simulink model "pmsm_2dof_control"  (R2018b)
settings: Solver=VariableStepAuto  StartTime=0.0  StopTime=20  RelTol=1e-3
model workspace (MATLAB code in the model file):
  | np=4; % pole pairs
  | phiv=0.1167; % rotor flux, wb
  | Kt=3/2*np*phiv;
  | f=7.43e-5; %Nm/(rad/s), friction
  | J=1.74e-4; %kgm*m, inertia
  | L=0.004; %H, inductance
  | Ld=L;
  | Lq=L;
  | Rs=1.74; %Ohm, armature resistance
  | Kp=50; % Prop gain in inner PI
  | Ki=2500; % I gain in inner PI
  | Ti = Kp/Ki;
  | h = 1e-2; % Sampling period
  | wN = pi/h; % Nyquist freq
  | wBf = 0.7*wN; % Cutoff freq for AA filter
  | w0f = wBf/2.11; % AA filter param
libraries: simulink x1
settings Model: Creator=kjartan  LastModifiedBy=kjartan

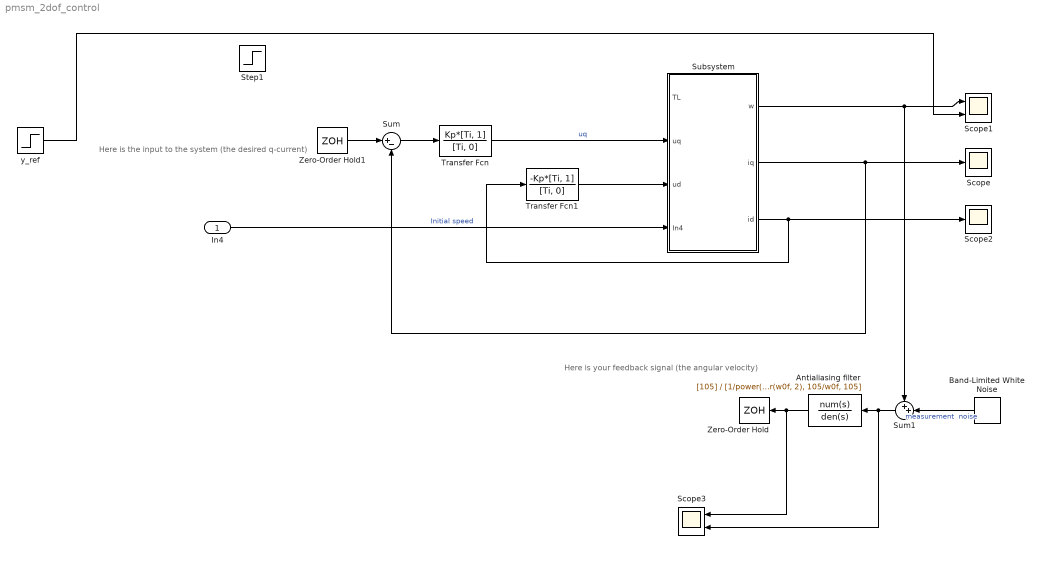
== system pmsm_2dof_control ==
  note: Here is the input to the system (the desired q-current)
  note: Here is your feedback signal (the angular velocity)
  In4 : Inport
  Antialiasing filter : TransferFcn  Numerator=[105]  Denominator=[1/power(w0f,4), 10/power(w0f, 3), 45/power(w0f, 2), 105/w0f, 105]
  Band-Limited White Noise : simulink/Sources/Band-Limited White Noise  Cov=1  Ts=h/10  seed=[23341]
  Scope : Scope
  Scope1 : Scope  NumInputPorts=2
  Scope2 : Scope
  Scope3 : Scope  NumInputPorts=2
  Step1 : Step  SampleTime=0
  Subsystem : Subsystem
  Sum : Sum  Inputs=|+-
  Sum1 : Sum  Inputs=++|
  Transfer Fcn : TransferFcn  Numerator=Kp*[Ti, 1]  Denominator=[Ti, 0]
  Transfer Fcn1 : TransferFcn  Numerator=-Kp*[Ti, 1]  Denominator=[Ti, 0]
  Zero-Order Hold : ZeroOrderHold  SampleTime=h
  Zero-Order Hold1 : ZeroOrderHold  SampleTime=h
  y_ref : Step  Time=0.2  After=10*2*pi  SampleTime=0
  wires:
  ? -> Subsystem/1(TL)  "load disturbance"
  Transfer Fcn/1 -> Subsystem/2(uq)  "uq"
  In4/1 -> Subsystem/4(In4)  "Initial speed"
  Subsystem/1(w) -> Scope1/1, Sum1/1
  Subsystem/2(iq) -> Sum/2, Scope/1
  Subsystem/3(id) -> Transfer Fcn1/1, Scope2/1
  Sum/1 -> Transfer Fcn/1
  Transfer Fcn1/1 -> Subsystem/3(ud)
  Antialiasing filter/1 -> Scope3/1, Zero-Order Hold/1
  Sum1/1 -> Scope3/2, Antialiasing filter/1
  Band-Limited White Noise/1 -> Sum1/2  "measurement  noise"
  Zero-Order Hold1/1 -> Sum/1
  y_ref/1 -> Scope1/2
  ? -> Zero-Order Hold1/1

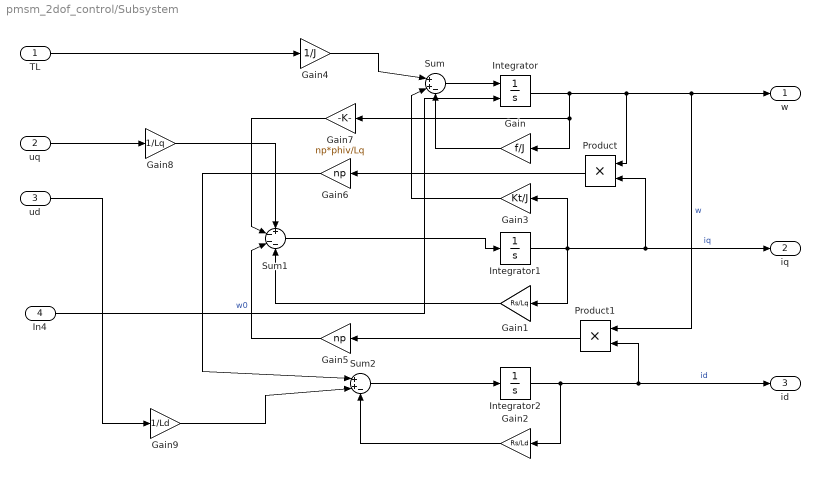
== system pmsm_2dof_control/Subsystem ==
  TL : Inport
  uq : Inport  Port=2
  ud : Inport  Port=3
  In4 : Inport  Port=4
  Gain : Gain  Gain=f/J
  Gain1 : Gain  Gain=Rs/Lq
  Gain2 : Gain  Gain=Rs/Ld
  Gain3 : Gain  Gain=Kt/J
  Gain4 : Gain  Gain=1/J
  Gain5 : Gain  Gain=np
  Gain6 : Gain  Gain=np
  Gain7 : Gain  Gain=np*phiv/Lq
  Gain8 : Gain  Gain=1/Lq
  Gain9 : Gain  Gain=1/Ld
  Integrator : Integrator  InitialConditionSource=external
  Integrator1 : Integrator
  Integrator2 : Integrator
  Product : Product
  Product1 : Product
  Sum : Sum  Inputs=|++-
  Sum1 : Sum  Inputs=+---
  Sum2 : Sum  Inputs=|++-
  w : Outport
  iq : Outport  Port=2
  id : Outport  Port=3
  wires:
  Product/1 -> Gain6/1
  Gain9/1 -> Sum2/2
  Gain2/1 -> Sum2/3
  Gain5/1 -> Sum1/3
  Gain/1 -> Sum/3
  Gain8/1 -> Sum1/1
  Product1/1 -> Gain5/1
  Gain3/1 -> Sum/2
  Gain7/1 -> Sum1/2
  In4/1 -> Integrator/2  "w0"
  Integrator1/1 -> Gain3/1, Gain1/1, iq/1, Product/2  "iq"
  uq/1 -> Gain8/1
  Sum1/1 -> Integrator1/1
  Integrator/1 -> Gain7/1, Gain/1, Product/1, w/1, Product1/1  "w"
  Gain6/1 -> Sum2/1
  Sum2/1 -> Integrator2/1
  Gain1/1 -> Sum1/4
  Integrator2/1 -> Gain2/1, id/1, Product1/2  "id"
  ud/1 -> Gain9/1
  Sum/1 -> Integrator/1
  TL/1 -> Gain4/1
  Gain4/1 -> Sum/1
